simulink model "sampleModel2063"  (R2023a)
settings: Solver=VariableStepAuto  StartTime=0.0  StopTime=10.0  RelTol=1e-3
libraries: hdlsllib x7, simulink x1
settings Model: Creator=user1  LastModifiedBy=user1

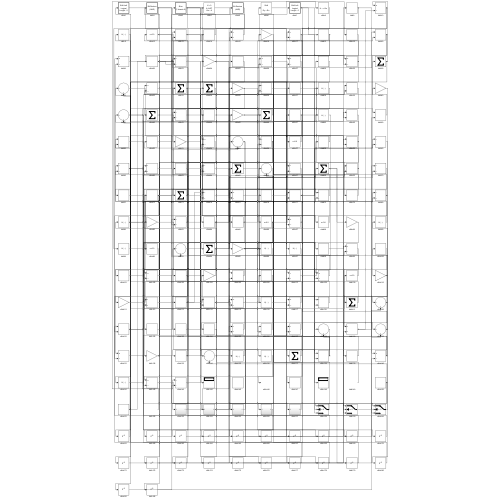
[thumbnail: Simulink's stored preview of the top-level diagram]
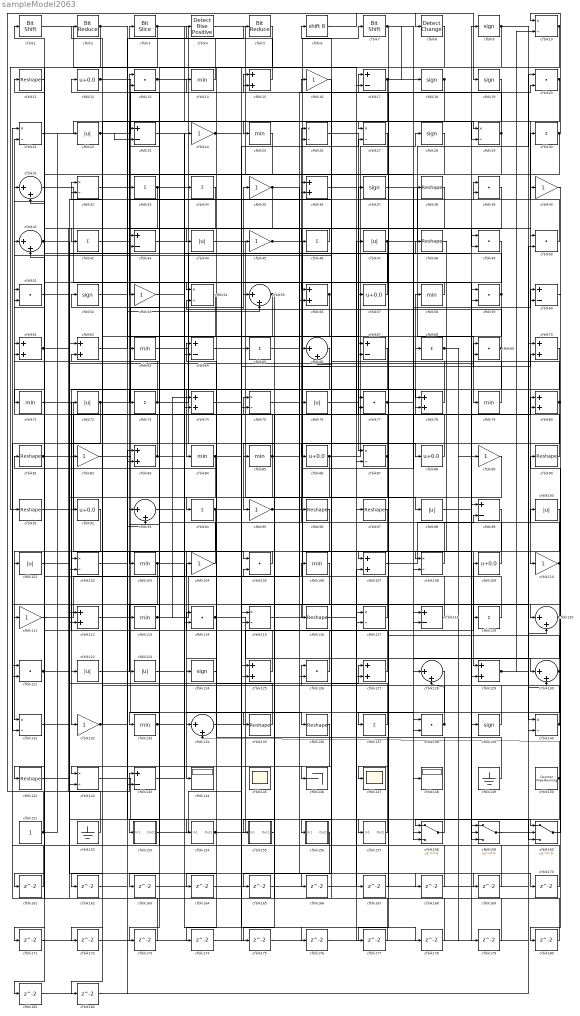
== system sampleModel2063 ==
  cfblk1 : hdlsllib/Logic and Bit Operations/Bit Shift  mode=Shift Left Logical  N=0
  cfblk{10,21,26..27,29,32,54,75,87,102,108,115,117,131,140,142} (16 alike) : Product  Inputs=*/  RndMeth=Zero  SaturateOnIntegerOverflow=on
  cfblk{22,44,47,72,76,98,100..101,122..123} (10 alike) : Abs  SaturateOnIntegerOverflow=off
  cfblk{14,25,58,63,71,79,84..85,103,106,113,133} (12 alike) : MinMax
  cfblk{16,24,35,40,45,53,82,89,95,104,110..111,132} (13 alike) : Gain
  cfblk{13,20,39,49..51,59,69,77,105,114,121,126,138} (14 alike) : DotProduct  OutDataTypeStr=Inherit: Inherit via internal rule
  cfblk{15,36,56,61..62,70,74,78,80,83,107,112,125,127,129} (15 alike) : Sum
  cfblk{12,57,86,88,92,109} (6 alike) : Bias  Bias=0.0  SaturateOnIntegerOverflow=off
  cfblk{11,38,48,81,90..91,96..97,116,135..136,141} (12 alike) : Reshape
  cfblk{17,23,43,60,64,67,99,118,143} (9 alike) : Sum  Inputs=+-
  cfblk{30,33..34,42,46,65,68,73,94,119,137} (11 alike) : Sum  Inputs=+
  cfblk{31,41,55,66,93,120,128,130,134} (9 alike) : Sum  Inputs=|++
  cfblk{9,18..19,28,37,52,124,139} (8 alike) : Signum
  cfblk144 : Display
  cfblk145 : Scope
      settings: Floating=on
  cfblk146 : Terminator
  cfblk147 : Scope
  cfblk148 : Display
  cfblk149 : Ground
  cfblk150 : hdlsllib/Sources/Counter Free-Running  NumBits=16  tsamp=-1
  cfblk151 : Constant  SampleTime=-1
  cfblk152 : Ground
  cfblk153 : Subsystem
      settings: LibrarySourceBlock=|
      | hdlsllib/Ports &
      | Subsystems/Subsystem
  cfblk154 : Subsystem
      settings: LibrarySourceBlock=|
      | hdlsllib/Ports &
      | Subsystems/Subsystem
  cfblk155 : Subsystem
      settings: LibrarySourceBlock=|
      | hdlsllib/Ports &
      | Subsystems/Subsystem
  cfblk156 : Subsystem
      settings: LibrarySourceBlock=|
      | hdlsllib/Ports &
      | Subsystems/Subsystem
  cfblk157 : Subsystem
      settings: LibrarySourceBlock=|
      | hdlsllib/Ports &
      | Subsystems/Subsystem
  cfblk158 : Switch  SaturateOnIntegerOverflow=off  InputSameDT=off
  cfblk159 : Switch  SaturateOnIntegerOverflow=off  InputSameDT=off
  cfblk160 : Switch  SaturateOnIntegerOverflow=off  InputSameDT=off
  cfblk{161..182} (22 alike) : Delay  SampleTime=1
  cfblk2 : hdlsllib/Logic and Bit Operations/Bit Reduce  mode=AND
  cfblk3 : hdlsllib/Logic and Bit Operations/Bit Slice  lidx=7  ridx=0
  cfblk4 : hdlsllib/Logic and Bit Operations/Detect Rise Positive  vinit=0  OutDataTypeStr=boolean
  cfblk5 : hdlsllib/Logic and Bit Operations/Bit Reduce  mode=AND
  cfblk6 : ArithShift  BitShiftNumber=8
  cfblk7 : hdlsllib/Logic and Bit Operations/Bit Shift  mode=Shift Left Logical  N=0
  cfblk8 : simulink/Logic and Bit Operations/Detect Change  vinit=0  OutDataTypeStr=boolean
      settings: LibrarySourceBlock=|
      | hdlsllib/Logic and Bit
      | Operations/Detect
      | Change
  wires:
  cfblk136/1 -> cfblk142/1
  cfblk7/1 -> cfblk18/1, cfblk57/1, cfblk159/2
  cfblk2/1 -> cfblk91/1, cfblk55/2, cfblk50/1
  cfblk68/1 -> cfblk89/1, cfblk179/1
  cfblk34/1 -> cfblk143/1
  cfblk92/1 -> cfblk132/1
  cfblk20/1 -> cfblk110/1, cfblk27/1
  cfblk115/1 -> cfblk7/1
  cfblk66/1 -> cfblk122/1
  cfblk139/1 -> cfblk126/1
  cfblk104/1 -> cfblk52/1
  cfblk142/1 -> cfblk160/1
  cfblk86/1 -> cfblk28/1, cfblk113/1, cfblk102/2
  cfblk67/1 -> cfblk84/1
  cfblk90/1 -> cfblk21/2
  cfblk158/1 -> cfblk16/1
  cfblk32/1 -> cfblk136/1
  cfblk45/1 -> cfblk98/1, cfblk59/2
  cfblk125/1 -> cfblk31/1
  cfblk108/1 -> cfblk26/1
  cfblk122/1 -> cfblk13/1
  cfblk149/1 -> cfblk81/1
  cfblk99/1 -> cfblk129/1
  cfblk13/1 -> cfblk95/1, cfblk15/2
  cfblk17/1 -> cfblk53/1, cfblk29/2
  cfblk154/1(Out1) -> cfblk109/1, cfblk27/2
  cfblk72/1 -> cfblk35/1, cfblk131/2, cfblk118/2
  cfblk50/1 -> cfblk30/1
  cfblk112/1 -> cfblk123/1
  cfblk97/1 -> cfblk131/1
  cfblk151/1 -> cfblk19/1, cfblk22/1
  cfblk43/1 -> cfblk128/1
  cfblk6/1 -> cfblk8/1
  cfblk141/1 -> cfblk127/1
  cfblk26/1 -> cfblk87/1
  cfblk76/1 -> cfblk37/1
  cfblk64/1 -> cfblk138/1
  cfblk37/1 -> cfblk79/1
  cfblk129/1 -> cfblk70/1, cfblk10/2
  cfblk71/1 -> cfblk105/1
  cfblk19/1 -> cfblk116/1
  cfblk35/1 -> cfblk153/1(In1), cfblk168/1
  cfblk59/1 -> cfblk11/1, cfblk172/1
  cfblk91/1 -> cfblk77/1
  cfblk109/1 -> cfblk12/1
  cfblk127/1 -> cfblk72/1
  cfblk118/1 -> cfblk51/1
  cfblk39/1 -> cfblk133/1
  cfblk114/1 -> cfblk130/1, cfblk67/2
  cfblk22/1 -> cfblk46/1, cfblk14/1, cfblk64/2, cfblk23/2
  cfblk93/1 -> cfblk34/1
  cfblk138/1 -> cfblk63/1, cfblk36/1, cfblk128/2
  cfblk79/1 -> cfblk33/1
  cfblk160/1 -> cfblk90/1
  cfblk8/1 -> cfblk103/1
  cfblk44/1 -> cfblk148/1
  cfblk42/1 -> cfblk139/1
  cfblk140/1 -> cfblk32/1, cfblk2/1
  cfblk82/1 -> cfblk144/1
  cfblk78/1 -> cfblk55/1
  cfblk155/1(Out1) -> cfblk75/1
  cfblk4/1 -> cfblk97/1
  cfblk111/1 -> cfblk104/1
  cfblk33/1 -> cfblk135/1, cfblk181/1
  cfblk88/1 -> cfblk58/1
  cfblk77/1 -> cfblk107/1, cfblk60/1, cfblk60/2
  cfblk153/1(Out1) -> cfblk65/1
  cfblk9/1 -> cfblk124/1, cfblk130/2
  cfblk123/1 -> cfblk39/1
  cfblk87/1 -> cfblk61/1, cfblk126/2
  cfblk46/1 -> cfblk44/1
  cfblk98/1 -> cfblk59/1
  cfblk117/1 -> cfblk93/1
  cfblk110/1 -> cfblk64/1, cfblk166/1
  cfblk31/1 -> cfblk83/2
  cfblk1/1 -> cfblk117/2
  cfblk12/1 -> cfblk127/2, cfblk67/1
  cfblk3/1 -> cfblk118/1, cfblk29/1, cfblk17/2, cfblk111/1
  cfblk57/1 -> cfblk6/1
  cfblk73/1 -> cfblk9/1, cfblk41/2
  cfblk152/1 -> cfblk61/2
  cfblk150/1 -> cfblk158/1, cfblk160/3, cfblk134/2
  cfblk102/1 -> cfblk157/1(In1)
  cfblk116/1 -> cfblk138/2
  cfblk18/1 -> cfblk42/1, cfblk96/1
  cfblk119/1 -> cfblk62/2
  cfblk40/1 -> cfblk120/1
  cfblk10/1 -> cfblk137/1, cfblk147/1
  cfblk56/1 -> cfblk92/1, cfblk163/1
  cfblk81/1 -> cfblk47/1, cfblk39/2
  cfblk27/1 -> cfblk146/1
  cfblk94/1 -> cfblk76/1, cfblk69/2, cfblk114/2
  cfblk21/1 -> cfblk25/1
  cfblk16/1 -> cfblk86/1
  cfblk105/1 -> cfblk102/1
  cfblk106/1 -> cfblk115/2
  cfblk58/1 -> cfblk56/1
  cfblk15/1 -> cfblk4/1
  cfblk62/1 -> cfblk5/1
  cfblk132/1 -> cfblk32/2, cfblk159/3
  cfblk29/1 -> cfblk141/1, cfblk15/1
  cfblk107/1 -> cfblk99/2
  cfblk69/1 -> cfblk85/1, cfblk54/2
  cfblk52/1 -> cfblk93/2
  cfblk63/1 -> cfblk75/2
  cfblk101/1 -> cfblk80/1
  cfblk55/1 -> cfblk155/1(In1), cfblk74/2
  cfblk95/1 -> cfblk140/1, cfblk38/1, cfblk108/2, cfblk159/1
  cfblk83/1 -> cfblk24/1, cfblk51/2
  cfblk89/1 -> cfblk134/1
  cfblk113/1 -> cfblk56/2, cfblk74/1
  cfblk121/1 -> cfblk69/1, cfblk78/2
  cfblk84/1 -> cfblk45/1, cfblk36/2, cfblk173/1
  cfblk133/1 -> cfblk80/2, cfblk23/1
  cfblk47/1 -> cfblk20/1, cfblk101/1
  cfblk143/1 -> cfblk40/1
  cfblk23/1 -> cfblk49/2
  cfblk135/1 -> cfblk114/1
  cfblk126/1 -> cfblk82/1
  cfblk28/1 -> cfblk71/1
  cfblk159/1 -> cfblk160/2
  cfblk41/1 -> cfblk78/1, cfblk154/1(In1)
  cfblk30/1 -> cfblk10/1, cfblk94/1
  cfblk24/1 -> cfblk158/2, cfblk87/2
  cfblk48/1 -> cfblk108/1
  cfblk49/1 -> cfblk54/1
  cfblk65/1 -> cfblk20/2
  cfblk120/1 -> cfblk119/1, cfblk158/3
  cfblk157/1(Out1) -> cfblk66/2
  cfblk61/1 -> cfblk88/1, cfblk43/2
  cfblk54/1 -> cfblk73/1
  cfblk137/1 -> cfblk106/1
  cfblk14/1 -> cfblk3/1
  cfblk96/1 -> cfblk142/2
  cfblk103/1 -> cfblk48/1, cfblk121/2
  cfblk85/1 -> cfblk43/1, cfblk112/2, cfblk68/1
  cfblk80/1 -> cfblk156/1(In1), cfblk41/1
  cfblk74/1 -> cfblk26/2
  cfblk75/1 -> cfblk70/2
  cfblk5/1 -> cfblk125/2
  cfblk130/1 -> cfblk17/1, cfblk100/1, cfblk175/1
  cfblk25/1 -> cfblk161/1
  cfblk161/1 -> cfblk21/1
  cfblk70/1 -> cfblk162/1
  cfblk162/1 -> cfblk143/2
  cfblk163/1 -> cfblk125/1
  cfblk128/1 -> cfblk164/1
  cfblk164/1 -> cfblk120/2
  cfblk156/1(Out1) -> cfblk165/1
  cfblk165/1 -> cfblk117/1
  cfblk166/1 -> cfblk99/1
  cfblk36/1 -> cfblk167/1
  cfblk167/1 -> cfblk77/2
  cfblk168/1 -> cfblk31/2
  cfblk131/1 -> cfblk169/1
  cfblk169/1 -> cfblk62/1
  cfblk51/1 -> cfblk170/1
  cfblk170/1 -> cfblk13/2
  cfblk11/1 -> cfblk171/1
  cfblk171/1 -> cfblk107/2
  cfblk172/1 -> cfblk129/2
  cfblk173/1 -> cfblk121/1
  cfblk124/1 -> cfblk174/1
  cfblk174/1 -> cfblk115/1
  cfblk175/1 -> cfblk140/2
  cfblk53/1 -> cfblk176/1
  cfblk176/1 -> cfblk49/1
  cfblk100/1 -> cfblk177/1
  cfblk177/1 -> cfblk112/1
  cfblk134/1 -> cfblk178/1
  cfblk178/1 -> cfblk1/1
  cfblk179/1 -> cfblk105/2
  cfblk60/1 -> cfblk180/1
  cfblk180/1 -> cfblk66/1
  cfblk181/1 -> cfblk50/2
  cfblk38/1 -> cfblk182/1
  cfblk182/1 -> cfblk83/1

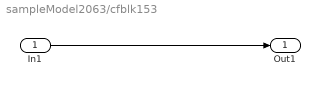
== system sampleModel2063/cfblk153 ==
  In1 : Inport
  Out1 : Outport
  wires:
  In1/1 -> Out1/1

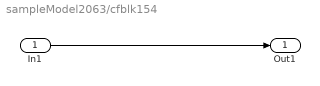
== system sampleModel2063/cfblk154 ==
  In1 : Inport
  Out1 : Outport
  wires:
  In1/1 -> Out1/1

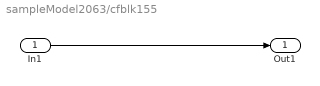
== system sampleModel2063/cfblk155 ==
  In1 : Inport
  Out1 : Outport
  wires:
  In1/1 -> Out1/1

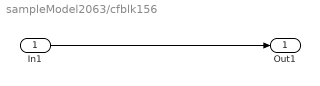
== system sampleModel2063/cfblk156 ==
  In1 : Inport
  Out1 : Outport
  wires:
  In1/1 -> Out1/1

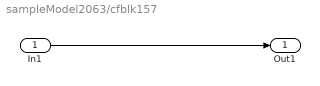
== system sampleModel2063/cfblk157 ==
  In1 : Inport
  Out1 : Outport
  wires:
  In1/1 -> Out1/1
